simulink model "pid_ecbf_sim_debug"  (R2021b)
settings: Solver=ode45  StartTime=0.0  StopTime=10.0  FixedStep=1e-3  RelTol=1e-3
PreLoadFcn:
  | acc = [0 0 0]
undefined symbols (not defined in the file or in its folder): P, pid_controller_debug
settings Model: Creator=USER  LastModifiedBy=an

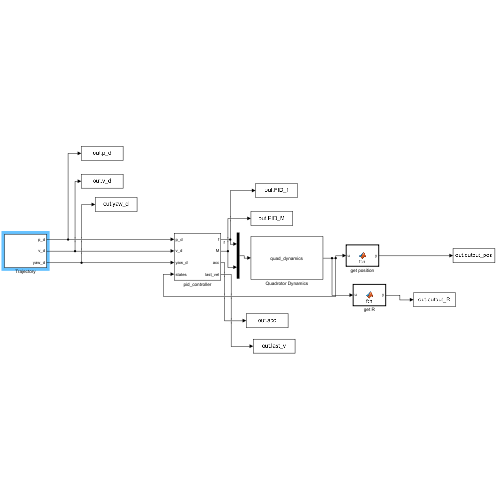
[thumbnail: Simulink's stored preview of the top-level diagram]
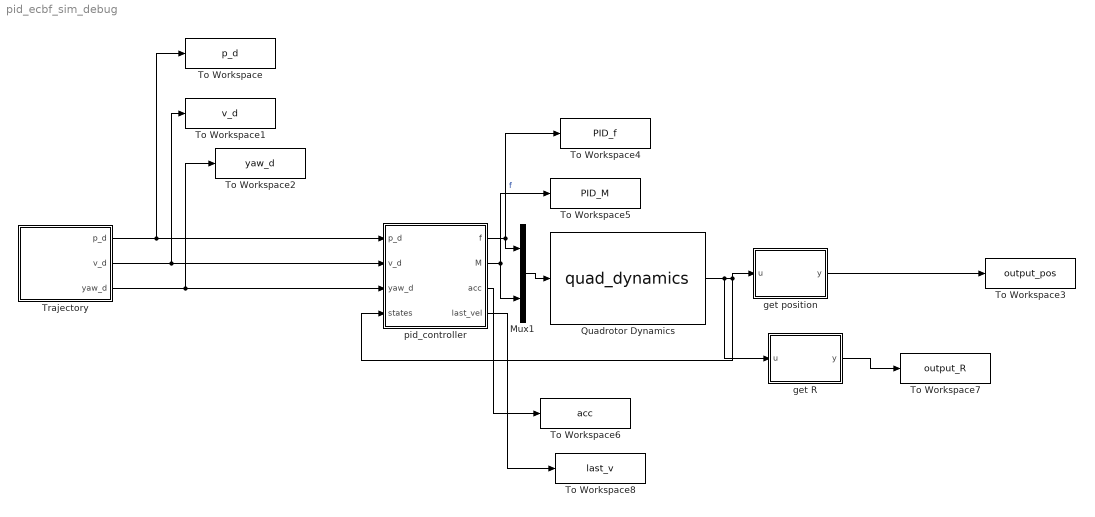
== system pid_ecbf_sim_debug ==
  Mux1 : Mux  Inputs=2
  Quadrotor Dynamics : S-Function  FunctionName=quad_dynamics  Parameters=P  SFunctionDeploymentMode=off  EnableBusSupport=off
  To Workspace : ToWorkspace  VariableName=p_d  SaveFormat=Timeseries  SampleTime=-1
  To Workspace1 : ToWorkspace  VariableName=v_d  SaveFormat=Timeseries  SampleTime=-1
  To Workspace2 : ToWorkspace  VariableName=yaw_d  SaveFormat=Timeseries  SampleTime=-1
  To Workspace3 : ToWorkspace  VariableName=output_pos  SaveFormat=Timeseries  SampleTime=-1
  To Workspace4 : ToWorkspace  VariableName=PID_f  SaveFormat=Timeseries  SampleTime=-1
  To Workspace5 : ToWorkspace  VariableName=PID_M  SaveFormat=Timeseries  SampleTime=-1
  To Workspace6 : ToWorkspace  VariableName=acc  SaveFormat=Timeseries  SampleTime=-1
  To Workspace7 : ToWorkspace  VariableName=output_R  SaveFormat=Timeseries  SampleTime=-1
  To Workspace8 : ToWorkspace  VariableName=last_v  SaveFormat=Timeseries  SampleTime=-1
  Trajectory : Subsystem
  get R : MATLAB Function  TreatAsAtomicUnit=on
  get position : MATLAB Function  TreatAsAtomicUnit=on
  pid_controller : Subsystem
  wires:
  Trajectory/1(p_d) -> To Workspace/1, pid_controller/1(p_d)
  Mux1/1 -> Quadrotor Dynamics/1
  pid_controller/1(f) -> Mux1/1, To Workspace4/1  "f"
  pid_controller/2(M) -> Mux1/2, To Workspace5/1
  Trajectory/3(yaw_d) -> To Workspace2/1, pid_controller/3(yaw_d)
  Quadrotor Dynamics/1 -> get R/1(u), get position/1(u), pid_controller/4(states)
  Trajectory/2(v_d) -> To Workspace1/1, pid_controller/2(v_d)
  get position/1(y) -> To Workspace3/1
  pid_controller/3(acc) -> To Workspace6/1
  get R/1(y) -> To Workspace7/1
  pid_controller/4(last_vel) -> To Workspace8/1

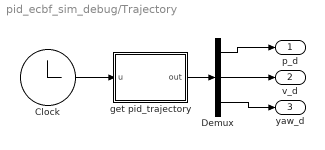
== system pid_ecbf_sim_debug/Trajectory ==
  Clock : Clock
  Demux : Demux  Outputs=3
  get pid_trajectory : MATLAB Function  TreatAsAtomicUnit=on
  p_d : Outport  PortDimensions=3  VectorParamsAs1DForOutWhenUnconnected=off
  v_d : Outport  Port=2  PortDimensions=3  VectorParamsAs1DForOutWhenUnconnected=off
  yaw_d : Outport  Port=3  PortDimensions=1  VectorParamsAs1DForOutWhenUnconnected=off
  wires:
  Clock/1 -> get pid_trajectory/1(u)
  Demux/1 -> p_d/1
  Demux/3 -> yaw_d/1
  Demux/2 -> v_d/1
  get pid_trajectory/1(out) -> Demux/1

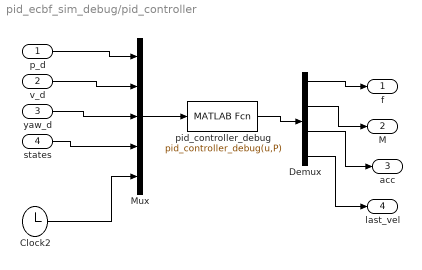
== system pid_ecbf_sim_debug/pid_controller ==
  p_d : Inport
  v_d : Inport  Port=2
  yaw_d : Inport  Port=3
  states : Inport  Port=4
  Clock2 : Clock
  Demux : Demux
  Mux : Mux  Inputs=5
  pid_controller_debug : MATLABFcn  MATLABFcn=pid_controller_debug(u,P)  OutputDimensions=10  SampleTime=P.Ts
  f : Outport  PortDimensions=1  VectorParamsAs1DForOutWhenUnconnected=off
  M : Outport  Port=2  PortDimensions=3  VectorParamsAs1DForOutWhenUnconnected=off
  acc : Outport  Port=3  PortDimensions=3  VectorParamsAs1DForOutWhenUnconnected=off
  last_vel : Outport  Port=4  PortDimensions=3  VectorParamsAs1DForOutWhenUnconnected=off
  wires:
  p_d/1 -> Mux/1
  Demux/1 -> f/1
  Demux/2 -> M/1
  states/1 -> Mux/4
  Clock2/1 -> Mux/5
  yaw_d/1 -> Mux/3
  v_d/1 -> Mux/2
  Mux/1 -> pid_controller_debug/1
  pid_controller_debug/1 -> Demux/1
  Demux/3 -> acc/1
  Demux/4 -> last_vel/1

== matlab function pid_ecbf_sim_debug/Trajectory/get pid_trajectory ==
  data: u input; out output
function out = pid_trajectory(u)

% input(1*1):time
% output(6*1):desired trajectory and desired yaw angle

t = u(end);
p_d = [1  1  -1.0];
v_d = [0.0  0.0  0.0]; 
yaw_d = 0.0;
out = [p_d v_d yaw_d];
end

== matlab function pid_ecbf_sim_debug/get R ==
  data: u input; y output
function y = fcn(u)

y = reshape(u(7:15),3,3);

== matlab function pid_ecbf_sim_debug/get position ==
  data: u input; y output
function y = fcn(u)

y = u(1:3);
